simulink model "cstr_sim"  (Simulink 6.6)
settings: Solver=ode45  StartTime=0  StopTime=24  RelTol=1e-3  AbsTol=1e-6
libraries: slident x3
settings Model: Creator=pelin  LastModifiedBy=rsingh
settings DebuggingCC: SignalResolutionControl=TryResolveAllWithWarning

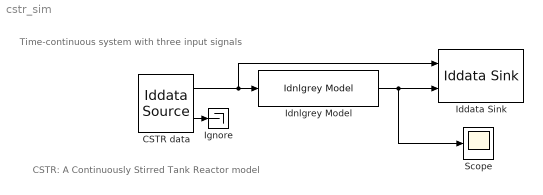
== system cstr_sim ==
  note: Time-continuous system with three input signals
  note: CSTR: A Continuously Stirred Tank Reactor model
  CSTR data : slident/Iddata Source  SystemSampleTime=-1  iddataobj=zv
  Iddata Sink : slident/Iddata Sink  SystemSampleTime=-1  datasetname=zsim  Ts=0.1  isu=off  isy=off
  Idnlgrey Model : slident/Idnlgrey Model  SystemSampleTime=-1  nlsys=nlgr  X0='m'
  Ignore : Terminator
  Scope : Scope
      settings: TimeRange=25  YMin=0  YMax=400
  wires:
  CSTR data/2 -> Ignore/1
  Idnlgrey Model/1 -> Iddata Sink/2, Scope/1
  CSTR data/1 -> Iddata Sink/1, Idnlgrey Model/1
